simulink model "dq_ABC_park"  (R2024b)
settings: Solver=VariableStepAuto  StartTime=0.0  StopTime=10.0  RelTol=1e-3
settings Model: Creator=罗芳成  LastModifiedBy=罗芳成

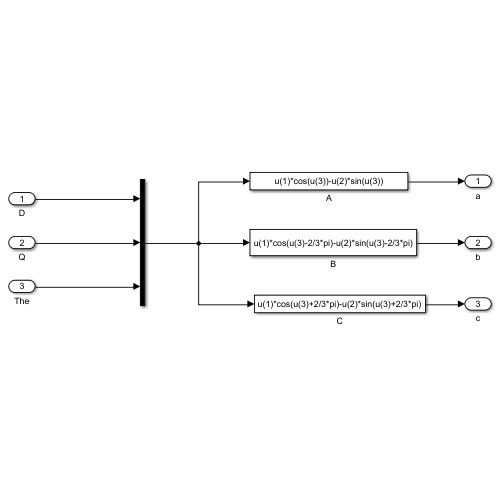
[thumbnail: Simulink's stored preview of the top-level diagram]
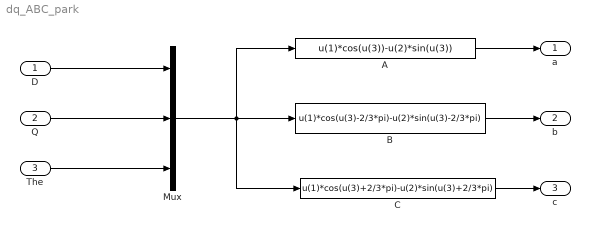
== system dq_ABC_park ==
  D : Inport
  Q : Inport  Port=2
  The : Inport  Port=3
  A : Fcn  Expr=u(1)*cos(u(3))-u(2)*sin(u(3))
  B : Fcn  Expr=u(1)*cos(u(3)-2/3*pi)-u(2)*sin(u(3)-2/3*pi)
  C : Fcn  Expr=u(1)*cos(u(3)+2/3*pi)-u(2)*sin(u(3)+2/3*pi)
  Mux : Mux  Inputs=3
  a : Outport
  b : Outport  Port=2
  c : Outport  Port=3
  wires:
  D/1 -> Mux/1
  Q/1 -> Mux/2
  The/1 -> Mux/3
  Mux/1 -> C/1, A/1, B/1
  A/1 -> a/1
  B/1 -> b/1
  C/1 -> c/1
